simulink model "CodeGenValidation"  (R2017a)
settings: Solver=VariableStepAuto  StartTime=0.0  StopTime=40  RelTol=1e-3
undefined symbols (not defined in the file or in its folder): Hz
settings Model: Creator=erich  LastModifiedBy=erich

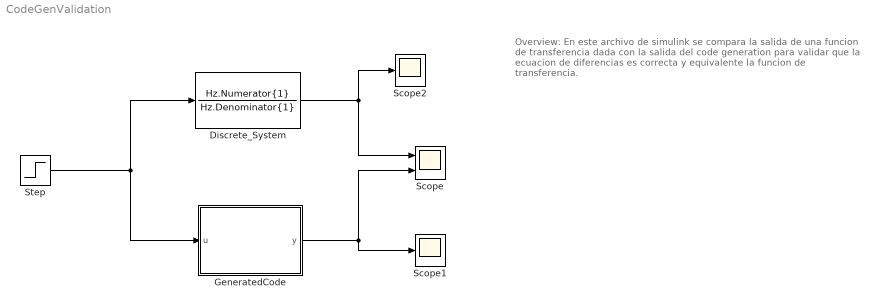
== system CodeGenValidation ==
  note: Overview:
      | En este archivo de simulink se compara la salida
      | de una funcion de transferencia dada con
      | la salida del code generation para validar que la
      | ecuacion de diferencias es correcta y equivalente
      | la funcion de transferencia.
  Discrete_System : DiscreteTransferFcn  Numerator=Hz.Numerator{1}  Denominator=Hz.Denominator{1}  SampleTime=.1
  GeneratedCode : MATLAB Function  TreatAsAtomicUnit=on  SystemSampleTime=.1
  Scope : Scope  NumInputPorts=2
  Scope1 : Scope
  Scope2 : Scope
  Step : Step  SampleTime=0
  wires:
  Step/1 -> Discrete_System/1, GeneratedCode/1(u)
  Discrete_System/1 -> Scope2/1, Scope/1
  GeneratedCode/1(y) -> Scope1/1, Scope/2

== matlab function CodeGenValidation/GeneratedCode ==
  data: u input; y output
function y = fcn(u)
persistent U;
if isempty(U)
	 U = zeros(1, 3);
end
persistent Y;
if isempty(Y)
	 Y = zeros(1, 2);
end
U = [u U(1:end-1)];
y_1 = (3867417694454701*U(2))/36028797018963968 - (6329353517423041*U(3))/72057594037927936 + (4389385923699487*Y(1))/2251799813685248 - (1070989120431317*Y(2))/1125899906842624;
Y = [y_1 Y(1:end-1)];
y = y_1;
